simulink model "psietesimulinkdiagrama"  (R2024b)
settings: Solver=VariableStepAuto  StartTime=0.0  StopTime=10.0  MaxStep=0.01  RelTol=1e-3
InitFcn:
  | R1=5000000;
  | R2=5000000;
  | R3=5000000;
  | C1=0.0000001;
  | C2=0.0000001;
  | u=5;

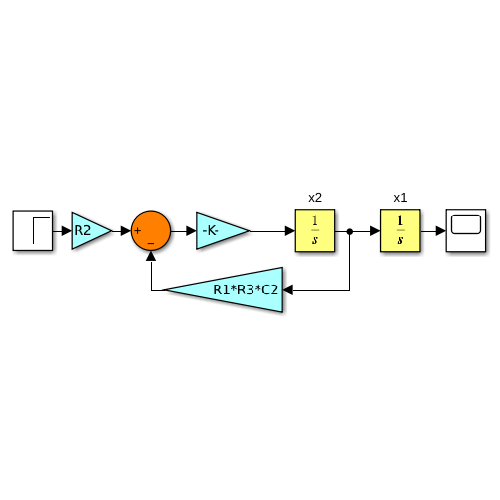
[thumbnail: Simulink's stored preview of the top-level diagram]
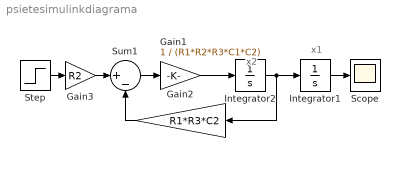
== system psietesimulinkdiagrama ==
  note: x2
  note: x1
  Gain1 : Gain  Gain=1 / (R1*R2*R3*C1*C2)
  Gain2 : Gain  Gain=R1*R3*C2
  Gain3 : Gain  Gain=R2
  Integrator1 : Integrator
  Integrator2 : Integrator
  Scope : Scope
  Step : Step  Time=0  After=5  SampleTime=0
  Sum1 : Sum  Inputs=|+-
  wires:
  Sum1/1 -> Gain1/1
  Gain1/1 -> Integrator2/1
  Integrator2/1 -> Integrator1/1, Gain2/1
  Gain2/1 -> Sum1/2
  Gain3/1 -> Sum1/1
  Step/1 -> Gain3/1
  Integrator1/1 -> Scope/1
